simulink model "CustomFuncBlock"  (R2015a)
settings: Solver=ode45  StartTime=0.0  StopTime=200  RelTol=1e-3
settings Model: Creator=Bilal  LastModifiedBy=Bilal

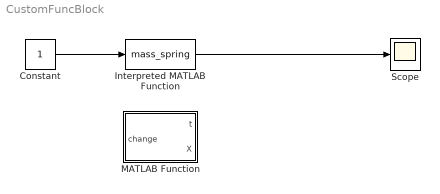
== system CustomFuncBlock ==
  Constant : Constant
  Interpreted MATLAB Function : MATLABFcn  MATLABFcn=mass_spring  Output1D=off
  MATLAB Function : MATLAB Function  TreatAsAtomicUnit=on
  Scope : Scope
  wires:
  Constant/1 -> Interpreted MATLAB Function/1
  Interpreted MATLAB Function/1 -> Scope/1
  ? -> MATLAB Function/1(change)

== matlab function CustomFuncBlock/MATLAB Function ==
  data: change input; t output; X output
function [t,X] = odeSolver(change)
%#codegen
X0=[0;0];% (Initial speed and position)
[t,X]=ode45(@(t,y)mass_spring(t,y,change),[0 200],X0);
